simulink model "RealLifeTrainModel"  (R2024a)
settings: Solver=ode1  StartTime=0.0  StopTime=Inf  FixedStep=0.001  RelTol=1e-3
PostLoadFcn:
  | , if any(exist('dsrtsu_mdlpostloadfcn', 'file') ~= 0), dsrtsu_mdlpostloadfcn('Execute', bdroot); end,
InitFcn:
  | , if any(exist('rtifpga_mdlclblib', 'file') ~= 0), rtifpga_mdlclblib('Init', bdroot); end,
undefined symbols (not defined in the file): DiscIntNeverNeededParam
libraries: deeplib x29, svdutilitieslib x28, simulink x8, eeGeneralControl x8, rti1202lib_adc_class1 x6, rti1202serlib x5, spsEdgeDetectorLib x5, rtiemclib x2, rti1202lib_dac_class1 x1
(part 2 of 8)

== system RealLifeTrainModel/CommSystem ==
  Fload : Inport
  dFload : Inport  Port=2
  Fhyd : Inport  Port=3
  dFhyd : Inport  Port=4
  Pa : Inport  Port=5
  Pb : Inport  Port=6
  X : Inport  Port=7
  dX : Inport  Port=8
  Ref : Inport  Port=9
  last_action : Inport  Port=10
  last_action_rl : Inport  Port=11
  last_action_control : Inport  Port=12
  Enable : EnablePort
  Constant : Constant
  If4 : If  IfExpression=u1 & 1
  IncSubSystem : Subsystem  TreatAsAtomicUnit=on
  ScopeCounter : Scope
  SendMessageSystem : Subsystem  TreatAsAtomicUnit=on
  wires:
  last_action_control/1 -> SendMessageSystem/12(last_action_control)
  X/1 -> SendMessageSystem/7(X)
  dFhyd/1 -> SendMessageSystem/4(dFhyd)
  Fhyd/1 -> SendMessageSystem/3(Fhyd)
  If4/2 -> IncSubSystem/Action
  last_action_rl/1 -> SendMessageSystem/11(last_action_rl)
  last_action/1 -> SendMessageSystem/10(last_action)
  dFload/1 -> SendMessageSystem/2(dFload)
  Fload/1 -> SendMessageSystem/1(Fload)
  Pa/1 -> SendMessageSystem/5(Pa)
  dX/1 -> SendMessageSystem/8(dX)
  Pb/1 -> SendMessageSystem/6(Pb)
  If4/1 -> SendMessageSystem/Action
  Ref/1 -> SendMessageSystem/9(Ref)
  Constant/1 -> If4/1

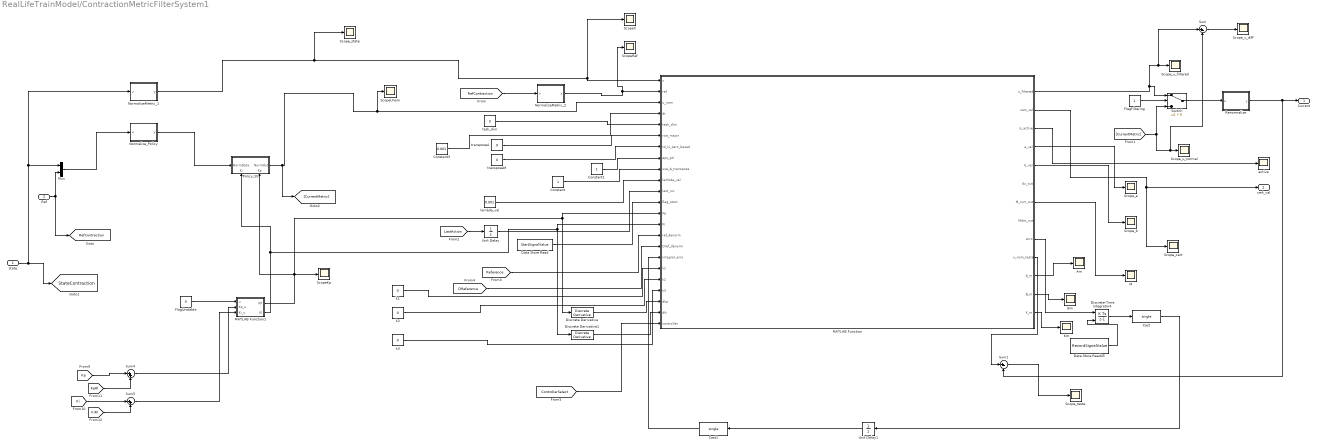
== system RealLifeTrainModel/ContractionMetricFilterSystem1 ==
  state : Inport
  Ref : Inport  Port=2
  Am : Scope
  Bm : Scope
  Cast : DataTypeConversion  OutDataTypeStr=single  SaturateOnIntegerOverflow=off  RndMeth=Floor
  Cast1 : DataTypeConversion  OutDataTypeStr=single  SaturateOnIntegerOverflow=off  RndMeth=Floor
  Constant : Constant
  Constant1 : Constant
  Constant3 : Constant  Value=0.001
  Data Store Read : DataStoreRead  DataStoreName=StartSignalValue  IndexOptions=Index vector (dialog)  Indices=1  OutputSizes=1
  Data Store Read45 : DataStoreRead  DataStoreName=RecordSignalValue  IndexOptions=Index vector (dialog)  Indices=1  OutputSizes=1
  Discrete Derivative : simulink/Discrete/Discrete Derivative  gainval=1.0  ICPrevScaledInput=0.0  OutMin=[]  OutMax=[]  OutDataType=fixdt(1, 16)  OutScaling=2^-10  DoSatur=off
  Discrete Derivative1 : simulink/Discrete/Discrete Derivative  gainval=1.0  ICPrevScaledInput=0.0  OutMin=[]  OutMax=[]  OutDataType=fixdt(1, 16)  OutScaling=2^-10  DoSatur=off
  Discrete-Time Integrator4 : DiscreteIntegrator  ExternalReset=falling  SampleTime=-1  ICPrevOutput=DiscIntNeverNeededParam  ICPrevScaledInput=DiscIntNeverNeededParam
  FlagFiltering : Constant
  FlagUnstable : Constant  Value=0
  Km : Scope
  M : Scope
  MATLAB Function : MATLAB Function  TreatAsAtomicUnit=on
  MATLAB Function1 : MATLAB Function  TreatAsAtomicUnit=on
  Mux : Mux  Inputs=2
  NormalizeMetric_1 : MATLAB Function  TreatAsAtomicUnit=on
  NormalizeMetric_2 : MATLAB Function  TreatAsAtomicUnit=on
  Normalize_Policy : MATLAB Function  TreatAsAtomicUnit=on
  Policy_SS : Subsystem
      settings: PortSchema="{\"entries\":[{\"content\":{\"sides\":[{\"content\":{\"connectorIds\":[\"In1\"]},\"type\":\"ConnectorPlacement.EquallySpacedRectSide\",\"uuid\":\"aff62fa4-063d-4c71-97b0-74a4cd3535bc\"},{\"content\":{\"connectorIds\":[\"Out1\"],\"side\":\"RIGHT\"},\"type\":\"ConnectorPlacement.EquallySpacedRectSide\",\"uuid\":\"01dd86b6-6835-48c6-94a2-7da686e8c645\"},{\"content\":{\"side\":\"TOP\"},\"type\":\"ConnectorPlacement.EquallySpacedRectSide\",\"uuid\":\"8b5720b6-3267-4312-8c98-f6d73204e352\"},{\"content\":{\"connectorIds\":[\"In2\",\"In3\"],\"side\":\"BOTTOM\"},\"type\":\"ConnectorPlacement.EquallySpacedRectSide\",\"uuid\":\"5afd0565-ca04-47d0-8ac2-f2d607cec9be\"}]},\"type\":\"ConnectorPlacement.EquallySpacedConnector\",\"uuid\":\"ef09f761-56e3-495c-a111-c24e12a3786f\"}],\"packageUris\":[\"http://schema.mathworks.com/mf0/Connector/R2020b\"],\"version\":\"1.0\"}"
  Renormalize : MATLAB Function  TreatAsAtomicUnit=on
  ScopeKp : Scope
  ScopeRef : Scope
  ScopeUnom : Scope
  ScopeX : Scope
  Scope_a : Scope
  Scope_b : Scope
  Scope_cert : Scope
  Scope_state : Scope
  Scope_teste : Scope
  Scope_u_diff : Scope
  Scope_u_filtered : Scope
  Scope_u_normal : Scope
  Sum : Sum  Inputs=|+-
  Sum1 : Sum  Inputs=|+-
  Sum4 : Sum  Inputs=|++
  Sum5 : Sum  Inputs=|++
  Switch : Switch  Criteria=u2 > Threshold  SaturateOnIntegerOverflow=off  InputSameDT=off
  Unit Delay : UnitDelay  SampleTime=-1  HasFrameUpgradeWarning=on
  Unit Delay1 : UnitDelay  SampleTime=-1  HasFrameUpgradeWarning=on
  active : Scope
  k1 : Constant  Value=0
  k2 : Constant  Value=0
  k3 : Constant  Value=0
  lambda_val : Constant  Value=0.001
  task_dim : Constant  Value=3
  transposeA : Constant  Value=0
  transposeM : Constant  Value=0
  Current : Outport
  cert_val : Outport  Port=2
  tag scope: RefContraction=global, StateContraction=global
  wires:
  Normalize_Policy/1(y) -> Policy_SS/1(NormData)
  Policy_SS/1(NormOut) -> [CurrentMetric], MATLAB Function/3(u_nom), ScopeUnom/1
  state/1 -> NormalizeMetric_1/1(u), Mux/1, [StateContraction]
  Ref/1 -> Mux/2, [RefContraction]
  Mux/1 -> Normalize_Policy/1(u)
  NormalizeMetric_1/1(y) -> Scope_state/1, ScopeX/1, MATLAB Function/1(x)
  [RefContraction] -> NormalizeMetric_2/1(u)
  NormalizeMetric_2/1(y) -> ScopeRef/1, MATLAB Function/2(ref)
  Renormalize/1(y) -> Sum1/2, Current/1
  MATLAB Function/2(cert_val) -> Scope_cert/1, cert_val/1
  MATLAB Function/3(is_active) -> active/1
  FlagFiltering/1 -> Switch/2
  MATLAB Function/1(u_filtered) -> Sum/1, Scope_u_filtered/1, Switch/1
  [CurrentMetric] -> Sum/2, Scope_u_normal/1, Switch/3
  Switch/1 -> Renormalize/1(u)
  Sum/1 -> Scope_u_diff/1
  MATLAB Function/4(a_val) -> Scope_a/1
  MATLAB Function/5(b_val) -> Scope_b/1
  Constant3/1 -> MATLAB Function/4(dt)
  task_dim/1 -> MATLAB Function/5(task_dim)
  transposeM/1 -> MATLAB Function/7(td_is_zero_based)
  lambda_val/1 -> MATLAB Function/10(lambda_val)
  [LastAction] -> Unit Delay/1
  Data Store Read/1 -> MATLAB Function/12(flag_start)
  MATLAB Function1/1(KP) -> MATLAB Function/13(Kp), Discrete Derivative/1, ScopeKp/1, Policy_SS/3(Kp)
  MATLAB Function1/2(KI) -> Policy_SS/2(Ki), MATLAB Function/14(Ki), Discrete Derivative1/1
  [Reference] -> MATLAB Function/15(ref_denorm)
  [DReference] -> MATLAB Function/16(Dref_denorm)
  Unit Delay/1 -> MATLAB Function/11(last_ixv)
  MATLAB Function/7(M_curr_out) -> M/1
  Data Store Read45/1 -> Discrete-Time Integrator4/2
  MATLAB Function/9(erro) -> Discrete-Time Integrator4/1
  Discrete-Time Integrator4/1 -> Cast/1
  Unit Delay1/1 -> Cast1/1
  Cast/1 -> Unit Delay1/1
  Cast1/1 -> MATLAB Function/17(integral_erro)
  MATLAB Function/10(u_nom_teste) -> Sum1/1
  Sum1/1 -> Scope_teste/1
  MATLAB Function/11(A_m) -> Am/1
  MATLAB Function/13(K_m) -> Km/1
  MATLAB Function/12(B_m) -> Bm/1
  Constant/1 -> MATLAB Function/9(use_A_transpose)
  Constant1/1 -> MATLAB Function/8(eps_pd)
  transposeA/1 -> MATLAB Function/6(row_major)
  k1/1 -> MATLAB Function/18(k1)
  k2/1 -> MATLAB Function/19(k2)
  k3/1 -> MATLAB Function/20(k3)
  [Kp] -> Sum4/1
  [Ki] -> Sum5/1
  [KiRl] -> Sum5/2
  [KpRl] -> Sum4/2
  Sum4/1 -> MATLAB Function1/2(Kp_s)
  Sum5/1 -> MATLAB Function1/3(Ki_s)
  FlagUnstable/1 -> MATLAB Function1/1(u)
  Discrete Derivative/1 -> MATLAB Function/21(dkp)
  Discrete Derivative1/1 -> MATLAB Function/22(dki)
  [ControllerSelect] -> MATLAB Function/23(controller)

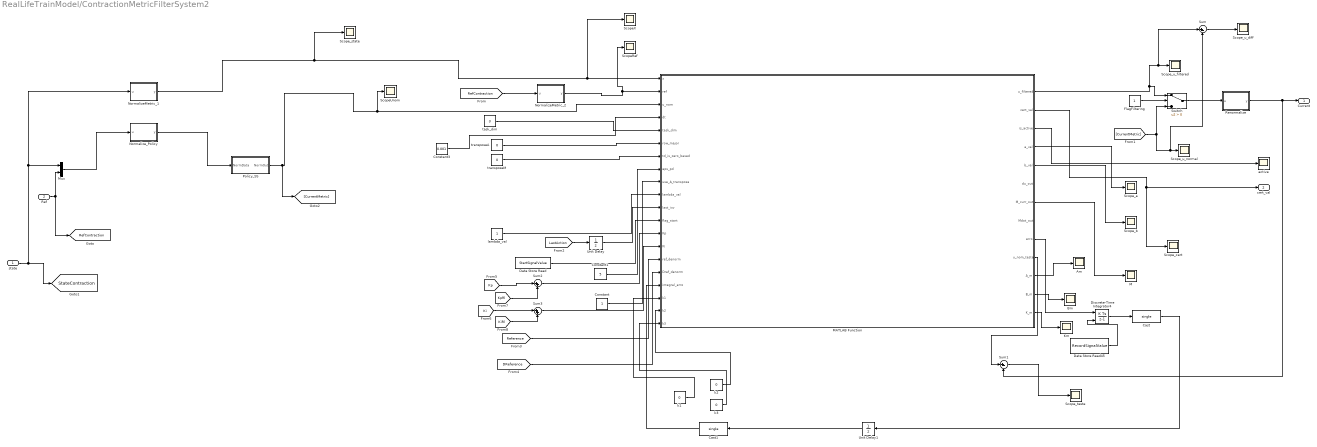
== system RealLifeTrainModel/ContractionMetricFilterSystem2 ==
  state : Inport
  Ref : Inport  Port=2
  Am : Scope
  Bm : Scope
  Cast : DataTypeConversion  OutDataTypeStr=single  SaturateOnIntegerOverflow=off  RndMeth=Floor
  Cast1 : DataTypeConversion  OutDataTypeStr=single  SaturateOnIntegerOverflow=off  RndMeth=Floor
  Constant : Constant
  Constant1 : Constant  Value=5
  Constant3 : Constant  Value=0.001
  Data Store Read : DataStoreRead  DataStoreName=StartSignalValue  IndexOptions=Index vector (dialog)  Indices=1  OutputSizes=1
  Data Store Read45 : DataStoreRead  DataStoreName=RecordSignalValue  IndexOptions=Index vector (dialog)  Indices=1  OutputSizes=1
  Discrete-Time Integrator4 : DiscreteIntegrator  ExternalReset=falling  SampleTime=-1  ICPrevOutput=DiscIntNeverNeededParam  ICPrevScaledInput=DiscIntNeverNeededParam
  FlagFiltering : Constant
  Km : Scope
  M : Scope
  MATLAB Function : MATLAB Function  TreatAsAtomicUnit=on
  Mux : Mux  Inputs=2
  NormalizeMetric_1 : MATLAB Function  TreatAsAtomicUnit=on
  NormalizeMetric_2 : MATLAB Function  TreatAsAtomicUnit=on
  Normalize_Policy : MATLAB Function  TreatAsAtomicUnit=on
  Policy_SS : Subsystem
  Renormalize : MATLAB Function  TreatAsAtomicUnit=on
  ScopeRef : Scope
  ScopeUnom : Scope
  ScopeX : Scope
  Scope_a : Scope
  Scope_b : Scope
  Scope_cert : Scope
  Scope_state : Scope
  Scope_teste : Scope
  Scope_u_diff : Scope
  Scope_u_filtered : Scope
  Scope_u_normal : Scope
  Sum : Sum  Inputs=|+-
  Sum1 : Sum  Inputs=|+-
  Sum2 : Sum  Inputs=|++
  Sum3 : Sum  Inputs=|++
  Switch : Switch  Criteria=u2 > Threshold  SaturateOnIntegerOverflow=off  InputSameDT=off
  Unit Delay : UnitDelay  SampleTime=-1  HasFrameUpgradeWarning=on
  Unit Delay1 : UnitDelay  SampleTime=-1  HasFrameUpgradeWarning=on
  active : Scope
  k1 : Constant  Value=0
  k2 : Constant  Value=0
  k3 : Constant  Value=0
  lambda_val : Constant
  task_dim : Constant  Value=3
  transposeA : Constant  Value=0
  transposeM : Constant  Value=0
  Current : Outport
  cert_val : Outport  Port=2
  tag scope: RefContraction=global, StateContraction=global
  wires:
  Normalize_Policy/1(y) -> Policy_SS/1(NormData)
  Policy_SS/1(NormOut) -> [CurrentMetric], MATLAB Function/3(u_nom), ScopeUnom/1
  state/1 -> NormalizeMetric_1/1(u), Mux/1, [StateContraction]
  Ref/1 -> Mux/2, [RefContraction]
  Mux/1 -> Normalize_Policy/1(u)
  NormalizeMetric_1/1(y) -> Scope_state/1, ScopeX/1, MATLAB Function/1(x)
  [RefContraction] -> NormalizeMetric_2/1(u)
  NormalizeMetric_2/1(y) -> ScopeRef/1, MATLAB Function/2(ref)
  Renormalize/1(y) -> Sum1/2, Current/1
  MATLAB Function/2(cert_val) -> Scope_cert/1, cert_val/1
  MATLAB Function/3(is_active) -> active/1
  FlagFiltering/1 -> Switch/2
  MATLAB Function/1(u_filtered) -> Sum/1, Scope_u_filtered/1, Switch/1
  [CurrentMetric] -> Sum/2, Scope_u_normal/1, Switch/3
  Switch/1 -> Renormalize/1(u)
  Sum/1 -> Scope_u_diff/1
  MATLAB Function/4(a_val) -> Scope_a/1
  MATLAB Function/5(b_val) -> Scope_b/1
  Constant3/1 -> MATLAB Function/4(dt)
  task_dim/1 -> MATLAB Function/5(task_dim)
  transposeM/1 -> MATLAB Function/7(td_is_zero_based)
  lambda_val/1 -> MATLAB Function/10(lambda_val)
  [LastAction] -> Unit Delay/1
  Data Store Read/1 -> MATLAB Function/12(flag_start)
  Sum2/1 -> MATLAB Function/13(Kp)
  Sum3/1 -> MATLAB Function/14(Ki)
  [Reference] -> MATLAB Function/15(ref_denorm)
  [DReference] -> MATLAB Function/16(Dref_denorm)
  [Kp] -> Sum2/1
  [Ki] -> Sum3/1
  [KpRl] -> Sum2/2
  [KiRl] -> Sum3/2
  Unit Delay/1 -> MATLAB Function/11(last_ixv)
  MATLAB Function/7(M_curr_out) -> M/1
  Data Store Read45/1 -> Discrete-Time Integrator4/2
  MATLAB Function/9(erro) -> Discrete-Time Integrator4/1
  Discrete-Time Integrator4/1 -> Cast/1
  Unit Delay1/1 -> Cast1/1
  Cast/1 -> Unit Delay1/1
  Cast1/1 -> MATLAB Function/17(integral_erro)
  MATLAB Function/10(u_nom_teste) -> Sum1/1
  Sum1/1 -> Scope_teste/1
  MATLAB Function/11(A_m) -> Am/1
  MATLAB Function/13(K_m) -> Km/1
  MATLAB Function/12(B_m) -> Bm/1
  Constant/1 -> MATLAB Function/9(use_A_transpose)
  Constant1/1 -> MATLAB Function/8(eps_pd)
  transposeA/1 -> MATLAB Function/6(row_major)
  k1/1 -> MATLAB Function/18(k1)
  k2/1 -> MATLAB Function/19(k2)
  k3/1 -> MATLAB Function/20(k3)

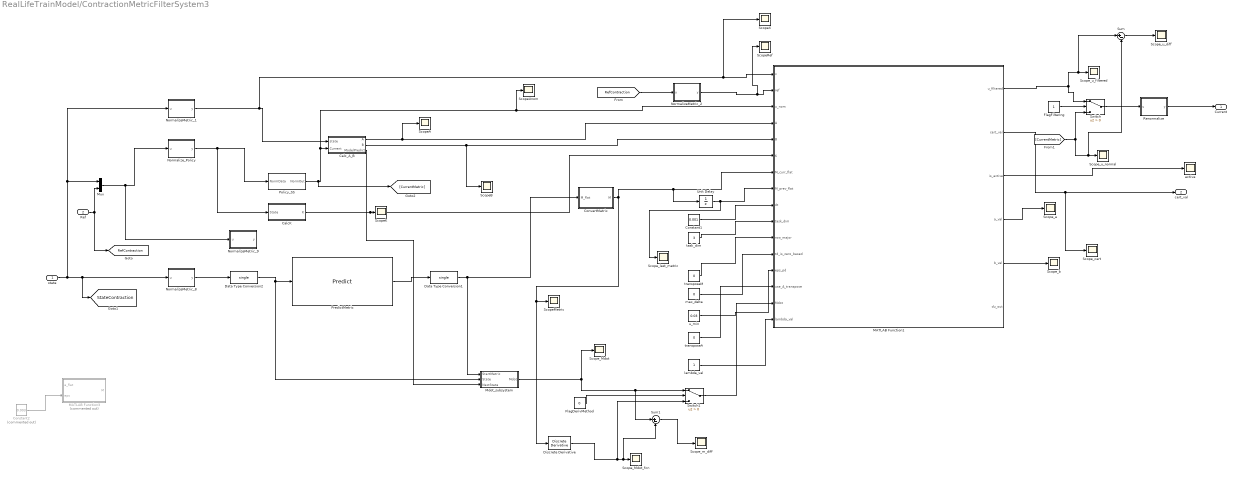
== system RealLifeTrainModel/ContractionMetricFilterSystem3 ==
  state : Inport
  Ref : Inport  Port=2
  CalcK : Subsystem
  Calc_A_B : Subsystem
  Constant1 : Constant  Value=0.001
  Constant2 : Constant  Commented=on  Value=0.003
  ConvertMatrix : MATLAB Function  TreatAsAtomicUnit=on
  Data Type Conversion1 : DataTypeConversion  OutDataTypeStr=single  SaturateOnIntegerOverflow=off  RndMeth=Floor
  Data Type Conversion2 : DataTypeConversion  OutDataTypeStr=single  SaturateOnIntegerOverflow=off  RndMeth=Floor
  Discrete Derivative : simulink/Discrete/Discrete Derivative  gainval=1.0  ICPrevScaledInput=0.0  OutMin=[]  OutMax=[]  OutDataType=fixdt(1, 16)  OutScaling=2^-10  DoSatur=off
  FlagDerivMethod : Constant  Value=0
  FlagFiltering : Constant
  MATLAB Function1 : MATLAB Function  TreatAsAtomicUnit=on
  MATLAB Function3 : MATLAB Function  Commented=on  TreatAsAtomicUnit=on
  Mdot_subsystem : Subsystem
  Mux : Mux  Inputs=2
  NormalizeMetric_1 : MATLAB Function  TreatAsAtomicUnit=on
  NormalizeMetric_2 : MATLAB Function  TreatAsAtomicUnit=on
  NormalizeMetric_8 : MATLAB Function  TreatAsAtomicUnit=on
  NormalizeMetric_9 : MATLAB Function  TreatAsAtomicUnit=on
  Normalize_Policy : MATLAB Function  TreatAsAtomicUnit=on
  Policy_SS : Subsystem
  PredictMetric : deeplib/Predict  Network=Network from MAT-file  NetworkFunction=squeezenet  NetworkFilePath=C:\Users\ic2d\Documents\GitHub\dSpace_Controllers_legged\metric.mat  MiniBatchSize=128  InputDataFormats={'input', 'BC';}  Predictions=on  Activations={}  ForceInterpretedSim=off  EnableDLNetwork=on  LastKnownNetworkFilePath='C:\Users\ic2d\Documents\GitHub\dSpace_Controllers_legged\metric.mat'  LastKnownNetworkTimeStamp=739864.429490740760229527950286865234375
  Renormalize : MATLAB Function  TreatAsAtomicUnit=on
  ScopeA : Scope
  ScopeB : Scope
  ScopeK : Scope
  ScopeMetric : Scope
  ScopeRef : Scope
  ScopeUnom : Scope
  ScopeX : Scope
  Scope_Mdot : Scope
  Scope_Mdot_fcn : Scope
  Scope_a : Scope
  Scope_b : Scope
  Scope_cert : Scope
  Scope_last_metric : Scope
  Scope_m_diff : Scope
  Scope_u_diff : Scope
  Scope_u_filtered : Scope
  Scope_u_normal : Scope
  Sum : Sum  Inputs=|+-
  Sum1 : Sum  Inputs=|+-
  Switch : Switch  Criteria=u2 > Threshold  SaturateOnIntegerOverflow=off  InputSameDT=off
  Switch1 : Switch  Criteria=u2 > Threshold  SaturateOnIntegerOverflow=off  InputSameDT=off
  Unit Delay : UnitDelay  SampleTime=-1  HasFrameUpgradeWarning=on
  active : Scope
  lambda_val : Constant
  max_delta : Constant  Value=0
  task_dim : Constant  Value=3
  transposeA : Constant  Value=0
  transposeM : Constant  Value=0
  u_min : Constant  Value=0.03
  Current : Outport
  cert_val : Outport  Port=2
  tag scope: RefContraction=global, StateContraction=global
  wires:
  Data Type Conversion2/1 -> Mdot_subsystem/2(State), PredictMetric/1
  Normalize_Policy/1(y) -> CalcK/1(State), Policy_SS/1(NormData)
  Policy_SS/1(NormOut) -> [CurrentMetric], ScopeUnom/1, MATLAB Function1/3(u_nom), Calc_A_B/2(Current)
  NormalizeMetric_8/1(y) -> Data Type Conversion2/1
  state/1 -> NormalizeMetric_1/1(u), Mux/1, [StateContraction], NormalizeMetric_8/1(u)
  Ref/1 -> Mux/2, [RefContraction]
  Mux/1 -> NormalizeMetric_9/1(u), Normalize_Policy/1(u)
  NormalizeMetric_1/1(y) -> ScopeX/1, MATLAB Function1/1(x), Calc_A_B/1(state)
  PredictMetric/1 -> Data Type Conversion1/1
  Constant1/1 -> MATLAB Function1/9(dt)
  u_min/1 -> MATLAB Function1/13(eps_pd)
  max_delta/1 -> MATLAB Function1/12(td_is_zero_based)
  lambda_val/1 -> MATLAB Function1/16(lambda_val)
  task_dim/1 -> MATLAB Function1/10(task_dim)
  [RefContraction] -> NormalizeMetric_2/1(u)
  NormalizeMetric_2/1(y) -> ScopeRef/1, MATLAB Function1/2(ref)
  Renormalize/1(y) -> Current/1
  MATLAB Function1/2(cert_val) -> Scope_cert/1, cert_val/1
  MATLAB Function1/3(is_active) -> active/1
  Data Type Conversion1/1 -> Mdot_subsystem/1(StartMetric), ConvertMatrix/1(M_flat)
  CalcK/1(K) -> MATLAB Function1/6(K), ScopeK/1
  Calc_A_B/1(A) -> MATLAB Function1/4(A), ScopeA/1
  FlagFiltering/1 -> Switch/2
  MATLAB Function1/1(u_filtered) -> Switch/1, Sum/1, Scope_u_filtered/1
  [CurrentMetric] -> Sum/2, Scope_u_normal/1, Switch/3
  Switch/1 -> Renormalize/1(u)
  Constant2/1 -> MATLAB Function3/2(eps)
  Sum/1 -> Scope_u_diff/1
  Calc_A_B/2(B) -> ScopeB/1, MATLAB Function1/5(B)
  MATLAB Function1/4(a_val) -> Scope_a/1
  MATLAB Function1/5(b_val) -> Scope_b/1
  Unit Delay/1 -> Scope_last_metric/1, MATLAB Function1/8(M_prev_flat)
  transposeA/1 -> MATLAB Function1/14(use_A_transpose)
  transposeM/1 -> MATLAB Function1/11(row_major)
  Calc_A_B/3(ModelPredict) -> Mdot_subsystem/3(NextState)
  Mdot_subsystem/1(Mdot) -> Scope_Mdot/1, Sum1/1, Switch1/1
  ConvertMatrix/1(M) -> Discrete Derivative/1, ScopeMetric/1, Unit Delay/1, MATLAB Function1/7(M_curr_flat)
  Discrete Derivative/1 -> Switch1/3, Sum1/2, Scope_Mdot_fcn/1
  Switch1/1 -> MATLAB Function1/15(Mdot)
  FlagDerivMethod/1 -> Switch1/2
  Sum1/1 -> Scope_m_diff/1

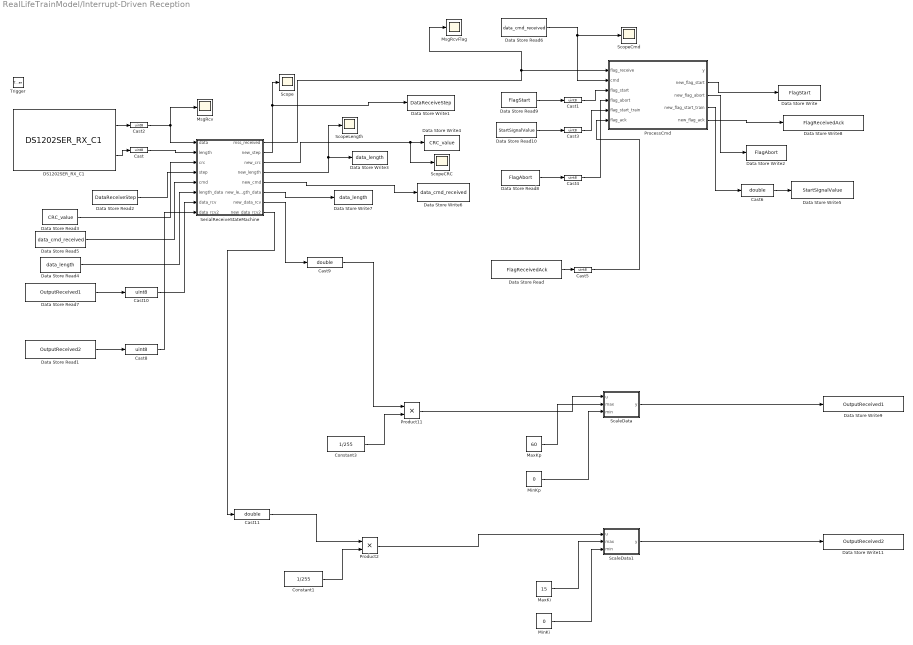
== system RealLifeTrainModel/Interrupt-Driven Reception ==
  Trigger : TriggerPort  TriggerType=function-call  VariantControl=Variant
  Cast{,1..5,8,10} (8 alike) : DataTypeConversion  OutDataTypeStr=uint8  SaturateOnIntegerOverflow=off  RndMeth=Floor
  Cast11 : DataTypeConversion  OutDataTypeStr=double  SaturateOnIntegerOverflow=off  RndMeth=Floor
  Cast6 : DataTypeConversion  OutDataTypeStr=double  SaturateOnIntegerOverflow=off  RndMeth=Floor
  Cast9 : DataTypeConversion  OutDataTypeStr=double  SaturateOnIntegerOverflow=off  RndMeth=Floor
  Constant1 : Constant  Value=1/255
  Constant3 : Constant  Value=1/255
  DS1202SER_RX_C1 : rti1202serlib/DS1202SER_RX_C1  Reserved1=[]  Reserved2=[]  Reserved3=[]  Reserved4=[]  DSProperties=struct('RTI',struct('IOBoardType',{{'DS1202','SER'}},'SlaveProcessor','NONE','Version',uint32(1),'BlockType',struct('isSLSource',uint8(1),'isSLSink',uint8(1),'isHWSource',uint8(0),'isHWSink',uint8(1),'isSetup',uint8(0),'isInline',uint8(1),'isNonInline',uint8(0),'isInterrupt',uint8(0),'isChannelwise',uint8(1)),'UnitType','GENSER','Identifier','RECEIVE','DialogType','ML','BlockSet','NONE'))  RTIBlockInterface=struct('BlockName',struct('Token',{{'DS1202SER_RX_C'}},'BlockParam',{{'ChannelNo'}}),'InputPortsWidth',int32(1),'InputPortsActive',0,'InputPortsDataType',{{'SS_UINT32'}},'InputPortsName',{{'NumBytes'}},'OutputPortsWidth',int32([7 1 1]),'OutputPortsActive',[1 1 0],'OutputPortsDataType',{{'SS_UINT8','SS_UINT32','SS_INT32'}},'OutputPortsName',{{'RXBytes','NumRXBytes','Status'}},'BlockDisplay',{{['Serial Receive'],'center'}},'IconTransparency','on','ParameterTunableNames',{{}},'InitLevel',2,'DialogFcn','guigenserreceive','MaskDescription',['To read data from the UART SW FIFO.'])  RTIBlockParameters=struct('BoardNo',{{1,'ON',[1 1]}},'ChannelNo',{{1,'ON',[1 2]}},'ChannelNumOf',{{2,'OFF',[]}},'ReceptionDataMode',{{1,'OFF',[]}},'ParamTunableMode',{{2,'OFF',[]}},'BytesRefNumOfT',{{'1','OFF',[1 inf]}},'BytesRefNumOfNT',{{'7','OFF',[1 inf]}},'BytesRefNumOfMax',{{'10','OFF',[1 inf]}},'BytesRefNumOfMode',{{0,'OFF',[]}},'BytesActNumOfMode',{{1,'OFF',[]}},'ReceptionStatusMode',{{0,'OFF',[]}},'FifoSizeDefault',{{64,'OFF',[]}},'TLCFileName',{{'rtigenserreceive','OFF',[]}})  RTISFcnParameters=struct('BoardNo','double','ChannelNo','double','ChannelNumOf','double','ReceptionDataMode','double','ParamTunableMode','double','BytesRefNumOfT','double','BytesRefNumOfNT','double','BytesRefNumOfMax','double','BytesRefNumOfMode','double','BytesActNumOfMode','double','ReceptionStatusMode','double','TLCFileName','char')  RTIBlockParaDefault=struct('BoardNo',1,'ChannelNo',1,'ChannelNumOf',2,'ReceptionDataMode',1,'ParamTunableMode',1,'BytesRefNumOfT',1,'BytesRefNumOfNT',1,'BytesRefNumOfMax',1,'BytesRefNumOfMode',0,'BytesActNumOfMode',1,'ReceptionStatusMode',1,'FifoSizeDefault',64,'TLCFileName','rtigenserreceive')
  Data Store Read : DataStoreRead  DataStoreName=FlagReceivedAck  IndexOptions=Index vector (dialog)  Indices=1  OutputSizes=1
  Data Store Read1 : DataStoreRead  DataStoreName=OutputReceived2  IndexOptions=Index vector (dialog)  Indices=1  OutputSizes=1
  Data Store Read10 : DataStoreRead  DataStoreName=StartSignalValue  IndexOptions=Index vector (dialog)  Indices=1  OutputSizes=1
  Data Store Read2 : DataStoreRead  DataStoreName=DataReceiveStep  IndexOptions=Index vector (dialog)  Indices=1  OutputSizes=1
  Data Store Read3 : DataStoreRead  DataStoreName=CRC_value  IndexOptions=Index vector (dialog)  Indices=1  OutputSizes=1
  Data Store Read4 : DataStoreRead  DataStoreName=data_length  IndexOptions=Index vector (dialog)  Indices=1  OutputSizes=1
  Data Store Read5 : DataStoreRead  DataStoreName=data_cmd_received  IndexOptions=Index vector (dialog)  Indices=1  OutputSizes=1
  Data Store Read6 : DataStoreRead  DataStoreName=data_cmd_received  IndexOptions=Index vector (dialog)  Indices=1  OutputSizes=1
  Data Store Read7 : DataStoreRead  DataStoreName=OutputReceived1  IndexOptions=Index vector (dialog)  Indices=1  OutputSizes=1
  Data Store Read8 : DataStoreRead  DataStoreName=FlagAbort  IndexOptions=Index vector (dialog)  Indices=1  OutputSizes=1
  Data Store Read9 : DataStoreRead  DataStoreName=FlagStart  IndexOptions=Index vector (dialog)  Indices=1  OutputSizes=1
  Data Store Write : DataStoreWrite  DataStoreName=FlagStart  IndexOptions=Index vector (dialog)  Indices=1  OutputSizes=1
  Data Store Write1 : DataStoreWrite  DataStoreName=DataReceiveStep  IndexOptions=Index vector (dialog)  Indices=1  OutputSizes=1
  Data Store Write11 : DataStoreWrite  DataStoreName=OutputReceived2  IndexOptions=Index vector (dialog)  Indices=1  OutputSizes=1
  Data Store Write2 : DataStoreWrite  DataStoreName=FlagAbort  IndexOptions=Index vector (dialog)  Indices=1  OutputSizes=1
  Data Store Write3 : DataStoreWrite  DataStoreName=data_length  IndexOptions=Index vector (dialog)  Indices=1  OutputSizes=1
  Data Store Write4 : DataStoreWrite  DataStoreName=CRC_value  IndexOptions=Index vector (dialog)  Indices=1  OutputSizes=1
  Data Store Write5 : DataStoreWrite  DataStoreName=StartSignalValue  IndexOptions=Index vector (dialog)  Indices=1  OutputSizes=1
  Data Store Write6 : DataStoreWrite  DataStoreName=data_cmd_received  IndexOptions=Index vector (dialog)  Indices=1  OutputSizes=1
  Data Store Write7 : DataStoreWrite  DataStoreName=data_length  IndexOptions=Index vector (dialog)  Indices=1  OutputSizes=1
  Data Store Write8 : DataStoreWrite  DataStoreName=FlagReceivedAck  IndexOptions=Index vector (dialog)  Indices=1  OutputSizes=1
  Data Store Write9 : DataStoreWrite  DataStoreName=OutputReceived1  IndexOptions=Index vector (dialog)  Indices=1  OutputSizes=1
  MaxKi : Constant  Value=15
  MaxKp : Constant  Value=60
  MinKi : Constant  Value=0
  MinKp : Constant  Value=0
  MsgRcv : Scope
  MsgRcvFlag : Scope
  ProcessCmd : MATLAB Function  TreatAsAtomicUnit=on
  Product11 : Product
  Product2 : Product
  ScaleData : MATLAB Function  TreatAsAtomicUnit=on
  ScaleData1 : MATLAB Function  TreatAsAtomicUnit=on
  Scope : Scope
  ScopeCRC : Scope
  ScopeCmd : Scope
  ScopeLength : Scope
  SerialReceiveStateMachine : MATLAB Function  TreatAsAtomicUnit=on
  wires:
  DS1202SER_RX_C1/1 -> Cast2/1
  SerialReceiveStateMachine/2(new_step) -> Scope/1, Data Store Write1/1
  Data Store Read2/1 -> SerialReceiveStateMachine/4(step)
  SerialReceiveStateMachine/4(new_length) -> ScopeLength/1, Data Store Write3/1
  SerialReceiveStateMachine/3(new_crc) -> ScopeCRC/1, Data Store Write4/1
  SerialReceiveStateMachine/1(mss_received) -> MsgRcvFlag/1, ProcessCmd/1(flag_receive)
  Data Store Read5/1 -> SerialReceiveStateMachine/5(cmd)
  Data Store Read4/1 -> SerialReceiveStateMachine/6(length_data)
  Data Store Read6/1 -> ProcessCmd/2(cmd), ScopeCmd/1
  SerialReceiveStateMachine/5(new_cmd) -> Data Store Write6/1
  SerialReceiveStateMachine/6(new_length_data) -> Data Store Write7/1
  ProcessCmd/2(new_flag_start) -> Data Store Write/1
  ProcessCmd/3(new_flag_abort) -> Data Store Write2/1
  ProcessCmd/4(new_flag_start_train) -> Cast6/1
  Data Store Read9/1 -> Cast1/1
  Data Store Read8/1 -> Cast4/1
  Data Store Read10/1 -> Cast3/1
  Data Store Read7/1 -> Cast10/1
  ProcessCmd/5(new_flag_ack) -> Data Store Write8/1
  Data Store Read/1 -> Cast5/1
  DS1202SER_RX_C1/2 -> Cast/1
  Cast/1 -> SerialReceiveStateMachine/2(length)
  Data Store Read3/1 -> SerialReceiveStateMachine/3(crc)
  Cast2/1 -> MsgRcv/1, SerialReceiveStateMachine/1(data)
  Cast1/1 -> ProcessCmd/3(flag_start)
  Cast3/1 -> ProcessCmd/5(flag_start_train)
  Cast4/1 -> ProcessCmd/4(flag_abort)
  Cast5/1 -> ProcessCmd/6(flag_ack)
  Cast6/1 -> Data Store Write5/1
  Constant3/1 -> Product11/2
  Cast9/1 -> Product11/1
  Cast10/1 -> SerialReceiveStateMachine/7(data_rcv)
  Data Store Read1/1 -> Cast8/1
  Cast8/1 -> SerialReceiveStateMachine/8(data_rcv2)
  SerialReceiveStateMachine/7(new_data_rcv) -> Cast9/1
  SerialReceiveStateMachine/8(new_data_rcv2) -> Cast11/1
  Cast11/1 -> Product2/1
  Constant1/1 -> Product2/2
  Product11/1 -> ScaleData/1(u)
  Product2/1 -> ScaleData1/1(u)
  MaxKp/1 -> ScaleData/2(max)
  MinKp/1 -> ScaleData/3(min)
  MaxKi/1 -> ScaleData1/2(max)
  MinKi/1 -> ScaleData1/3(min)
  ScaleData/1(y) -> Data Store Write9/1
  ScaleData1/1(y) -> Data Store Write11/1

== system RealLifeTrainModel/PolyDerivativeSubSystem1 ==
  Signal : Inport
  N : Inport  Port=2
  Constant : Constant  Value=0.001
  MATLAB Function : MATLAB Function  TreatAsAtomicUnit=on
  Mux : Mux  Inputs=40
  Unit Delay{1..39} (39 alike) : UnitDelay  SampleTime=-1  HasFrameUpgradeWarning=on
  dSignal : Outport
  ddSignal : Outport  Port=2
  dddSignal : Outport  Port=3
  wires:
  MATLAB Function/1(dx) -> dSignal/1
  Constant/1 -> MATLAB Function/2(Ts)
  Unit Delay12/1 -> Mux/5, Unit Delay13/1
  Unit Delay13/1 -> Mux/6, Unit Delay14/1
  Unit Delay9/1 -> Mux/2, Unit Delay10/1
  Unit Delay10/1 -> Mux/3, Unit Delay11/1
  Unit Delay11/1 -> Unit Delay12/1, Mux/4
  Signal/1 -> Mux/1, Unit Delay9/1
  Unit Delay15/1 -> Unit Delay16/1, Mux/8
  Unit Delay14/1 -> Mux/7, Unit Delay15/1
  Unit Delay16/1 -> Mux/9, Unit Delay1/1
  Unit Delay1/1 -> Unit Delay2/1, Mux/10
  Mux/1 -> MATLAB Function/1(k)
  Unit Delay2/1 -> Mux/11, Unit Delay3/1
  Unit Delay3/1 -> Mux/12, Unit Delay4/1
  Unit Delay4/1 -> Mux/13, Unit Delay5/1
  Unit Delay5/1 -> Mux/14, Unit Delay6/1
  Unit Delay6/1 -> Mux/15, Unit Delay7/1
  Unit Delay7/1 -> Unit Delay8/1, Mux/16
  Unit Delay8/1 -> Mux/17, Unit Delay17/1
  Unit Delay17/1 -> Mux/18, Unit Delay18/1
  Unit Delay18/1 -> Mux/19, Unit Delay19/1
  MATLAB Function/2(ddx) -> ddSignal/1
  MATLAB Function/3(dddx) -> dddSignal/1
  Unit Delay19/1 -> Unit Delay20/1, Mux/20
  Unit Delay20/1 -> Unit Delay21/1, Mux/21
  Unit Delay21/1 -> Unit Delay22/1, Mux/22
  Unit Delay22/1 -> Unit Delay23/1, Mux/23
  Unit Delay23/1 -> Unit Delay24/1, Mux/24
  Unit Delay24/1 -> Mux/25, Unit Delay25/1
  Unit Delay25/1 -> Unit Delay26/1, Mux/26
  Unit Delay26/1 -> Unit Delay27/1, Mux/27
  Unit Delay27/1 -> Unit Delay28/1, Mux/28
  Unit Delay28/1 -> Unit Delay29/1, Mux/29
  Unit Delay29/1 -> Unit Delay30/1, Mux/30
  Unit Delay30/1 -> Unit Delay31/1, Mux/31
  Unit Delay31/1 -> Unit Delay32/1, Mux/32
  Unit Delay32/1 -> Unit Delay33/1, Mux/33
  Unit Delay33/1 -> Unit Delay34/1, Mux/34
  Unit Delay34/1 -> Unit Delay35/1, Mux/35
  Unit Delay35/1 -> Unit Delay36/1, Mux/36
  Unit Delay36/1 -> Unit Delay37/1, Mux/37
  Unit Delay37/1 -> Unit Delay38/1, Mux/38
  Unit Delay38/1 -> Unit Delay39/1, Mux/39
  Unit Delay39/1 -> Mux/40
  N/1 -> MATLAB Function/3(n_points)

== system RealLifeTrainModel/PolyDerivativeSubSystem2 ==
  Signal : Inport
  N : Inport  Port=2
  Constant : Constant  Value=0.001
  MATLAB Function : MATLAB Function  TreatAsAtomicUnit=on
  Mux : Mux  Inputs=40
  Unit Delay{1..39} (39 alike) : UnitDelay  SampleTime=-1  HasFrameUpgradeWarning=on
  dSignal : Outport
  ddSignal : Outport  Port=2
  dddSignal : Outport  Port=3
  wires:
  MATLAB Function/1(dx) -> dSignal/1
  Constant/1 -> MATLAB Function/2(Ts)
  Unit Delay12/1 -> Mux/5, Unit Delay13/1
  Unit Delay13/1 -> Mux/6, Unit Delay14/1
  Unit Delay9/1 -> Mux/2, Unit Delay10/1
  Unit Delay10/1 -> Mux/3, Unit Delay11/1
  Unit Delay11/1 -> Unit Delay12/1, Mux/4
  Signal/1 -> Mux/1, Unit Delay9/1
  Unit Delay15/1 -> Unit Delay16/1, Mux/8
  Unit Delay14/1 -> Mux/7, Unit Delay15/1
  Unit Delay16/1 -> Mux/9, Unit Delay1/1
  Unit Delay1/1 -> Unit Delay2/1, Mux/10
  Mux/1 -> MATLAB Function/1(k)
  Unit Delay2/1 -> Mux/11, Unit Delay3/1
  Unit Delay3/1 -> Mux/12, Unit Delay4/1
  Unit Delay4/1 -> Mux/13, Unit Delay5/1
  Unit Delay5/1 -> Mux/14, Unit Delay6/1
  Unit Delay6/1 -> Mux/15, Unit Delay7/1
  Unit Delay7/1 -> Unit Delay8/1, Mux/16
  Unit Delay8/1 -> Mux/17, Unit Delay17/1
  Unit Delay17/1 -> Mux/18, Unit Delay18/1
  Unit Delay18/1 -> Mux/19, Unit Delay19/1
  MATLAB Function/2(ddx) -> ddSignal/1
  MATLAB Function/3(dddx) -> dddSignal/1
  Unit Delay19/1 -> Unit Delay20/1, Mux/20
  Unit Delay20/1 -> Unit Delay21/1, Mux/21
  Unit Delay21/1 -> Unit Delay22/1, Mux/22
  Unit Delay22/1 -> Unit Delay23/1, Mux/23
  Unit Delay23/1 -> Unit Delay24/1, Mux/24
  Unit Delay24/1 -> Mux/25, Unit Delay25/1
  Unit Delay25/1 -> Unit Delay26/1, Mux/26
  Unit Delay26/1 -> Unit Delay27/1, Mux/27
  Unit Delay27/1 -> Unit Delay28/1, Mux/28
  Unit Delay28/1 -> Unit Delay29/1, Mux/29
  Unit Delay29/1 -> Unit Delay30/1, Mux/30
  Unit Delay30/1 -> Unit Delay31/1, Mux/31
  Unit Delay31/1 -> Unit Delay32/1, Mux/32
  Unit Delay32/1 -> Unit Delay33/1, Mux/33
  Unit Delay33/1 -> Unit Delay34/1, Mux/34
  Unit Delay34/1 -> Unit Delay35/1, Mux/35
  Unit Delay35/1 -> Unit Delay36/1, Mux/36
  Unit Delay36/1 -> Unit Delay37/1, Mux/37
  Unit Delay37/1 -> Unit Delay38/1, Mux/38
  Unit Delay38/1 -> Unit Delay39/1, Mux/39
  Unit Delay39/1 -> Mux/40
  N/1 -> MATLAB Function/3(n_points)

== system RealLifeTrainModel/PolyDerivativeSubSystem3 ==
  Signal : Inport
  N : Inport  Port=2
  Constant : Constant  Value=0.001
  MATLAB Function : MATLAB Function  TreatAsAtomicUnit=on
  Mux : Mux  Inputs=40
  Unit Delay{1..39} (39 alike) : UnitDelay  SampleTime=-1  HasFrameUpgradeWarning=on
  dSignal : Outport
  ddSignal : Outport  Port=2
  dddSignal : Outport  Port=3
  wires:
  MATLAB Function/1(dx) -> dSignal/1
  Constant/1 -> MATLAB Function/2(Ts)
  Unit Delay12/1 -> Mux/5, Unit Delay13/1
  Unit Delay13/1 -> Mux/6, Unit Delay14/1
  Unit Delay9/1 -> Mux/2, Unit Delay10/1
  Unit Delay10/1 -> Mux/3, Unit Delay11/1
  Unit Delay11/1 -> Unit Delay12/1, Mux/4
  Signal/1 -> Mux/1, Unit Delay9/1
  Unit Delay15/1 -> Unit Delay16/1, Mux/8
  Unit Delay14/1 -> Mux/7, Unit Delay15/1
  Unit Delay16/1 -> Mux/9, Unit Delay1/1
  Unit Delay1/1 -> Unit Delay2/1, Mux/10
  Mux/1 -> MATLAB Function/1(k)
  Unit Delay2/1 -> Mux/11, Unit Delay3/1
  Unit Delay3/1 -> Mux/12, Unit Delay4/1
  Unit Delay4/1 -> Mux/13, Unit Delay5/1
  Unit Delay5/1 -> Mux/14, Unit Delay6/1
  Unit Delay6/1 -> Mux/15, Unit Delay7/1
  Unit Delay7/1 -> Unit Delay8/1, Mux/16
  Unit Delay8/1 -> Mux/17, Unit Delay17/1
  Unit Delay17/1 -> Mux/18, Unit Delay18/1
  Unit Delay18/1 -> Mux/19, Unit Delay19/1
  MATLAB Function/2(ddx) -> ddSignal/1
  MATLAB Function/3(dddx) -> dddSignal/1
  Unit Delay19/1 -> Unit Delay20/1, Mux/20
  Unit Delay20/1 -> Unit Delay21/1, Mux/21
  Unit Delay21/1 -> Unit Delay22/1, Mux/22
  Unit Delay22/1 -> Unit Delay23/1, Mux/23
  Unit Delay23/1 -> Unit Delay24/1, Mux/24
  Unit Delay24/1 -> Mux/25, Unit Delay25/1
  Unit Delay25/1 -> Unit Delay26/1, Mux/26
  Unit Delay26/1 -> Unit Delay27/1, Mux/27
  Unit Delay27/1 -> Unit Delay28/1, Mux/28
  Unit Delay28/1 -> Unit Delay29/1, Mux/29
  Unit Delay29/1 -> Unit Delay30/1, Mux/30
  Unit Delay30/1 -> Unit Delay31/1, Mux/31
  Unit Delay31/1 -> Unit Delay32/1, Mux/32
  Unit Delay32/1 -> Unit Delay33/1, Mux/33
  Unit Delay33/1 -> Unit Delay34/1, Mux/34
  Unit Delay34/1 -> Unit Delay35/1, Mux/35
  Unit Delay35/1 -> Unit Delay36/1, Mux/36
  Unit Delay36/1 -> Unit Delay37/1, Mux/37
  Unit Delay37/1 -> Unit Delay38/1, Mux/38
  Unit Delay38/1 -> Unit Delay39/1, Mux/39
  Unit Delay39/1 -> Mux/40
  N/1 -> MATLAB Function/3(n_points)

== system RealLifeTrainModel/PolyDerivativeSubSystem4 ==
  Signal : Inport
  Constant : Constant  Value=0.001
  MATLAB Function : MATLAB Function  TreatAsAtomicUnit=on
  Mux : Mux  Inputs=20
  Unit Delay{1..18} (18 alike) : UnitDelay  SampleTime=-1  HasFrameUpgradeWarning=on
  dSignal : Outport
  ddSignal : Outport  Port=2
  dddSignal : Outport  Port=3
  wires:
  MATLAB Function/1(dx) -> dSignal/1
  Constant/1 -> MATLAB Function/2(Ts)
  Unit Delay12/1 -> Mux/5, Unit Delay13/1
  Unit Delay13/1 -> Mux/6, Unit Delay14/1
  Unit Delay9/1 -> Mux/2, Unit Delay10/1
  Unit Delay10/1 -> Mux/3, Unit Delay11/1
  Unit Delay11/1 -> Unit Delay12/1, Mux/4
  Signal/1 -> Unit Delay9/1, Mux/1
  Unit Delay15/1 -> Unit Delay16/1, Mux/8
  Unit Delay14/1 -> Mux/7, Unit Delay15/1
  Unit Delay16/1 -> Unit Delay1/1, Mux/9
  Unit Delay1/1 -> Unit Delay2/1, Mux/10
  Mux/1 -> MATLAB Function/1(k)
  Unit Delay2/1 -> Unit Delay3/1, Mux/11
  Unit Delay3/1 -> Unit Delay4/1, Mux/12
  Unit Delay4/1 -> Unit Delay5/1, Mux/13
  Unit Delay5/1 -> Unit Delay6/1, Mux/14
  Unit Delay6/1 -> Unit Delay7/1, Mux/15
  Unit Delay7/1 -> Unit Delay8/1, Mux/16
  Unit Delay8/1 -> Unit Delay17/1, Mux/17
  Unit Delay17/1 -> Unit Delay18/1, Mux/18
  Unit Delay18/1 -> Mux/20, Mux/19
  MATLAB Function/2(ddx) -> ddSignal/1
  MATLAB Function/3(dddx) -> dddSignal/1

== system RealLifeTrainModel/PolyDerivativeSubSystem5 ==
  Signal : Inport
  N : Inport  Port=2
  Constant : Constant  Value=0.001
  MATLAB Function : MATLAB Function  TreatAsAtomicUnit=on
  Mux : Mux  Inputs=40
  Unit Delay{1..39} (39 alike) : UnitDelay  SampleTime=-1  HasFrameUpgradeWarning=on
  dSignal : Outport
  ddSignal : Outport  Port=2
  dddSignal : Outport  Port=3
  wires:
  MATLAB Function/1(dx) -> dSignal/1
  Constant/1 -> MATLAB Function/2(Ts)
  Unit Delay12/1 -> Mux/5, Unit Delay13/1
  Unit Delay13/1 -> Mux/6, Unit Delay14/1
  Unit Delay9/1 -> Mux/2, Unit Delay10/1
  Unit Delay10/1 -> Mux/3, Unit Delay11/1
  Unit Delay11/1 -> Unit Delay12/1, Mux/4
  Signal/1 -> Mux/1, Unit Delay9/1
  Unit Delay15/1 -> Unit Delay16/1, Mux/8
  Unit Delay14/1 -> Mux/7, Unit Delay15/1
  Unit Delay16/1 -> Mux/9, Unit Delay1/1
  Unit Delay1/1 -> Unit Delay2/1, Mux/10
  Mux/1 -> MATLAB Function/1(k)
  Unit Delay2/1 -> Mux/11, Unit Delay3/1
  Unit Delay3/1 -> Mux/12, Unit Delay4/1
  Unit Delay4/1 -> Mux/13, Unit Delay5/1
  Unit Delay5/1 -> Mux/14, Unit Delay6/1
  Unit Delay6/1 -> Mux/15, Unit Delay7/1
  Unit Delay7/1 -> Unit Delay8/1, Mux/16
  Unit Delay8/1 -> Mux/17, Unit Delay17/1
  Unit Delay17/1 -> Mux/18, Unit Delay18/1
  Unit Delay18/1 -> Mux/19, Unit Delay19/1
  MATLAB Function/2(ddx) -> ddSignal/1
  MATLAB Function/3(dddx) -> dddSignal/1
  Unit Delay19/1 -> Unit Delay20/1, Mux/20
  Unit Delay20/1 -> Unit Delay21/1, Mux/21
  Unit Delay21/1 -> Unit Delay22/1, Mux/22
  Unit Delay22/1 -> Unit Delay23/1, Mux/23
  Unit Delay23/1 -> Unit Delay24/1, Mux/24
  Unit Delay24/1 -> Mux/25, Unit Delay25/1
  Unit Delay25/1 -> Unit Delay26/1, Mux/26
  Unit Delay26/1 -> Unit Delay27/1, Mux/27
  Unit Delay27/1 -> Unit Delay28/1, Mux/28
  Unit Delay28/1 -> Unit Delay29/1, Mux/29
  Unit Delay29/1 -> Unit Delay30/1, Mux/30
  Unit Delay30/1 -> Unit Delay31/1, Mux/31
  Unit Delay31/1 -> Unit Delay32/1, Mux/32
  Unit Delay32/1 -> Unit Delay33/1, Mux/33
  Unit Delay33/1 -> Unit Delay34/1, Mux/34
  Unit Delay34/1 -> Unit Delay35/1, Mux/35
  Unit Delay35/1 -> Unit Delay36/1, Mux/36
  Unit Delay36/1 -> Unit Delay37/1, Mux/37
  Unit Delay37/1 -> Unit Delay38/1, Mux/38
  Unit Delay38/1 -> Unit Delay39/1, Mux/39
  Unit Delay39/1 -> Mux/40
  N/1 -> MATLAB Function/3(n_points)

== system RealLifeTrainModel/PolyDerivativeSubSystem6 ==
  Signal : Inport
  Constant : Constant  Value=0.001
  MATLAB Function : MATLAB Function  TreatAsAtomicUnit=on
  Mux : Mux  Inputs=20
  Unit Delay{1..18} (18 alike) : UnitDelay  SampleTime=-1  HasFrameUpgradeWarning=on
  dSignal : Outport
  ddSignal : Outport  Port=2
  dddSignal : Outport  Port=3
  wires:
  MATLAB Function/1(dx) -> dSignal/1
  Constant/1 -> MATLAB Function/2(Ts)
  Unit Delay12/1 -> Mux/5, Unit Delay13/1
  Unit Delay13/1 -> Mux/6, Unit Delay14/1
  Unit Delay9/1 -> Mux/2, Unit Delay10/1
  Unit Delay10/1 -> Mux/3, Unit Delay11/1
  Unit Delay11/1 -> Unit Delay12/1, Mux/4
  Signal/1 -> Unit Delay9/1, Mux/1
  Unit Delay15/1 -> Unit Delay16/1, Mux/8
  Unit Delay14/1 -> Mux/7, Unit Delay15/1
  Unit Delay16/1 -> Unit Delay1/1, Mux/9
  Unit Delay1/1 -> Unit Delay2/1, Mux/10
  Mux/1 -> MATLAB Function/1(k)
  Unit Delay2/1 -> Unit Delay3/1, Mux/11
  Unit Delay3/1 -> Unit Delay4/1, Mux/12
  Unit Delay4/1 -> Unit Delay5/1, Mux/13
  Unit Delay5/1 -> Unit Delay6/1, Mux/14
  Unit Delay6/1 -> Unit Delay7/1, Mux/15
  Unit Delay7/1 -> Unit Delay8/1, Mux/16
  Unit Delay8/1 -> Unit Delay17/1, Mux/17
  Unit Delay17/1 -> Unit Delay18/1, Mux/18
  Unit Delay18/1 -> Mux/20, Mux/19
  MATLAB Function/2(ddx) -> ddSignal/1
  MATLAB Function/3(dddx) -> dddSignal/1

== system RealLifeTrainModel/RTI Data ==
  RTI Data Store : Subsystem  Tag="struct('public',struct('sub',struct('name',{{'Teste_PID'}},'data',{{struct('TH',struct('thTaskInfo',struct('taskType',{'TIMER','HWINT','TMRINT','SWINT','GLINT'},'tasksNumOf',{1,1,0,0,0},'srcIds',{{'TIMERA'},{'UART_EVENTS_CH1_INT0'},{},{},{}},'taskNames',{{['Timer Task 1']},{'DS1202SER_INT_C1_I1'},{},{},{}})),'th_tc',struct('dataType',{'TASK','TASK'},'taskGroupId',{'',''},'taskGroupList',{{},{}},'taskSchedulingPolicy',{'FCFS','FCFS'},'taskType',{'TIMER','HWINT'},'blkh',{-1,'Teste_PID/DS1202SER_INT_C1_I1'},'srcId',{'TIMERA','UART_EVENTS_CH1_INT0'},'srcSgnName',{['Timer A interrupt'],['UART Ch1 RX SW FIFO interrupt']},'srcCpuName',{'',''},'taskName',{['Timer Task 1  [0.001] s'],'DS1202SER_INT_C1_I1'},'taskNameDisplayExt',{'',''},'smplTime',{0.001,0},'smplTimeOffs',{0,0},'hasFixedPriority',{0,0},'priority',{2,1},'hasFixedOvc',{0,0},'ovcType',{1,3},'ovcMax',{1,1}),'tc_th',struct('dataType',{'TASK','TASK'},'taskGroupId',{'',''},'taskGroupList',{{},{}},'taskSchedulingPolicy',{'FCFS','FCFS'},'taskType',{'TIMER','HWINT'},'blkh',{-1,'Teste_PID/DS1202SER_INT_C1_I1'},'srcId',{'TIMERA','UART_EVENTS_CH1_INT0'},'srcSgnName',{['Timer A interrupt'],['UART Ch1 RX SW FIFO interrupt']},'srcCpuName',{'',''},'taskName',{['Timer Task 1  [0.001] s'],'DS1202SER_INT_C1_I1'},'taskNameDisplayExt',{'',''},'smplTime',{0.001,0},'smplTimeOffs',{0,0},'hasFixedPriority',{0,0},'priority',{2,1},'hasFixedOvc',{0,0},'ovcType',{1,3},'ovcMax',{1,1}))}})),'private',struct('version',struct('dsVer',uint32(2)),'access',struct('type','Model','isPerm',1)))"  mask(RTI_DATA_STORE){}
      mask help:
      | RTI Data Store Block. This block is used by RTI to store internal model dependent data. Deleting this block will result in data loss.
      |
      | NEVER DELETE, COPY, OR MODIFY THIS BLOCK!
      mask Help:
      | RTI Data Store Block. This block is used by RTI to store internal model dependent data. Deleting this block will result in data loss.
      | 
      | NEVER DELETE, COPY, OR MODIFY THIS BLOCK!
      mask Display: text(0.5, 0.5, ' ', 'HorizontalAlignment', 'center');

== system RealLifeTrainModel/CommSystem/IncSubSystem ==
  Input : Inport
  Action Port : ActionPort  ActionPortLabel=else
  Constant : Constant
  Sum : Sum  Inputs=|++
  Out1 : Outport
  wires:
  Input/1 -> Sum/1
  Constant/1 -> Sum/2
  Sum/1 -> Out1/1

== system RealLifeTrainModel/CommSystem/SendMessageSystem ==
  Fload : Inport
  dFload : Inport  Port=2
  Fhyd : Inport  Port=3
  dFhyd : Inport  Port=4
  Pa : Inport  Port=5
  Pb : Inport  Port=6
  X : Inport  Port=7
  dX : Inport  Port=8
  Ref : Inport  Port=9
  last_action : Inport  Port=10
  last_action_rl : Inport  Port=11
  last_action_control : Inport  Port=12
  Action Port : ActionPort  ActionPortLabel=if(u1 & 1)
  AND1 : Logic  IconShape=distinctive  AllPortsSameDT=off  OutDataTypeStr=boolean
  AND2 : Logic  Inputs=3  IconShape=distinctive  AllPortsSameDT=off  OutDataTypeStr=boolean
  CancelSubsystem : Subsystem  TreatAsAtomicUnit=on
  Data Store Memory : DataStoreMemory  DataStoreName=CancelCounter  WriteAfterWriteMsg=warning  ShowAdditionalParam=off
  Data Store Memory1 : DataStoreMemory  DataStoreName=CancelLimit  WriteAfterWriteMsg=warning  InitialValue=7  ShowAdditionalParam=off
  Data Store Read : DataStoreRead  DataStoreName=StartSignalValue  IndexOptions=Index vector (dialog)  Indices=1  OutputSizes=1
  Data Store Read1 : DataStoreRead  DataStoreName=FlagReceivedAck  IndexOptions=Index vector (dialog)  Indices=1  OutputSizes=1
  Data Store Read2 : DataStoreRead  DataStoreName=CancelCounter  IndexOptions=Index vector (dialog)  Indices=1  OutputSizes=1
  Data Store Read3 : DataStoreRead  DataStoreName=CancelLimit  IndexOptions=Index vector (dialog)  Indices=1  OutputSizes=1
  Data Store Read6 : DataStoreRead  DataStoreName=FlagAbort  IndexOptions=Index vector (dialog)  Indices=1  OutputSizes=1
  Data Store Read7 : DataStoreRead  DataStoreName=StartSignalValue  IndexOptions=Index vector (dialog)  Indices=1  OutputSizes=1
  Data Store Read8 : DataStoreRead  DataStoreName=FlagAbort  IndexOptions=Index vector (dialog)  Indices=1  OutputSizes=1
  If Action Subsystem : Subsystem  TreatAsAtomicUnit=on
  If Action Subsystem1 : Subsystem  TreatAsAtomicUnit=on
  If2 : If  IfExpression="u1  == 1"
  If3 : If  IfExpression="u1  == 1"
  NOT1 : Logic  Operator=NOT  IconShape=distinctive  AllPortsSameDT=off  OutDataTypeStr=boolean
  NOT2 : Logic  Operator=NOT  IconShape=distinctive  AllPortsSameDT=off  OutDataTypeStr=boolean
  OR : Logic  Operator=OR  IconShape=distinctive  AllPortsSameDT=off  OutDataTypeStr=boolean
  ScopeFlagAck : Scope
  ScopeFlagStartTrain : Scope
  SendObs : Subsystem  TreatAsAtomicUnit=on
  SendObs1 : Subsystem  Commented=on  TreatAsAtomicUnit=on
  wires:
  Data Store Read6/1 -> OR/2
  OR/1 -> If2/1
  AND2/1 -> If3/1
  If3/1 -> SendObs/Action
  Data Store Read7/1 -> AND2/2
  If2/2 -> If Action Subsystem/Action
  If Action Subsystem/1(Out1) -> AND2/1
  Data Store Read8/1 -> NOT2/1
  AND1/1 -> OR/1
  Data Store Read1/1 -> ScopeFlagAck/1, NOT1/1
  NOT2/1 -> AND2/3
  NOT1/1 -> AND1/1
  If2/1 -> CancelSubsystem/Action
  Data Store Read/1 -> AND1/2, ScopeFlagStartTrain/1
  If3/2 -> If Action Subsystem1/Action
  Fload/1 -> SendObs/1(Fload)
  dFload/1 -> SendObs/2(dFload)
  Fhyd/1 -> SendObs/3(Fhyd)
  dFhyd/1 -> SendObs/4(dFhyd)
  Pa/1 -> SendObs/5(Pa)
  Pb/1 -> SendObs/6(Pb)
  X/1 -> SendObs/7(X)
  dX/1 -> SendObs/8(dX)
  Ref/1 -> SendObs/9(Ref)
  last_action/1 -> SendObs/10(last_action)
  last_action_rl/1 -> SendObs/11(last_action_rl)
  last_action_control/1 -> SendObs/12(last_action_control)
  Data Store Read2/1 -> CancelSubsystem/1(CancelCounter)
  Data Store Read3/1 -> CancelSubsystem/2(CancelLimit)

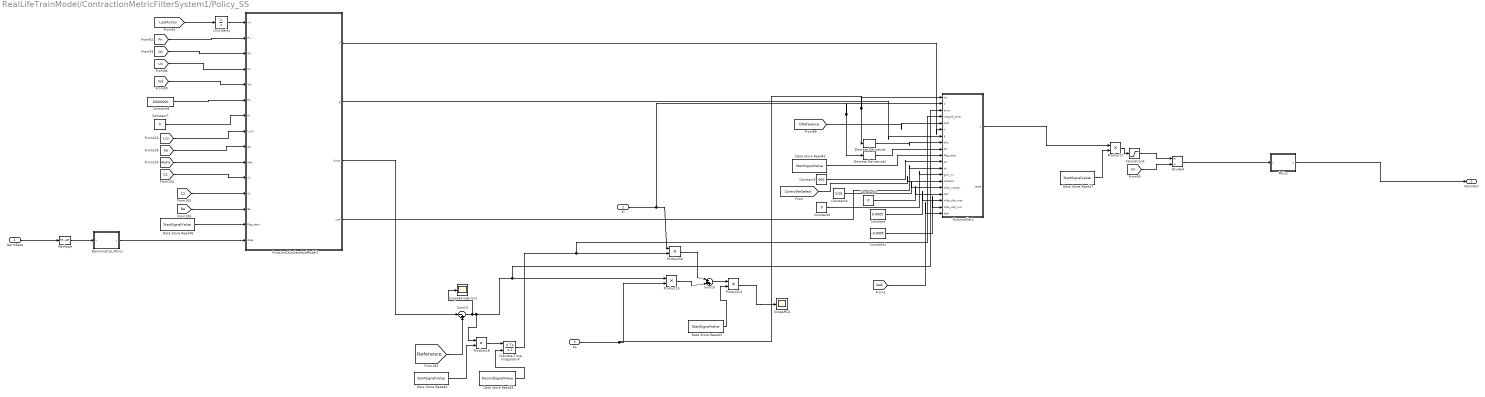
== system RealLifeTrainModel/ContractionMetricFilterSystem1/Policy_SS ==
  NormData : Inport
  Ki : Inport  Port=2
  Kp : Inport  Port=3
  Constant : Constant  Value=0.0005
  Constant1 : Constant  Value=-0.0005
  Constant3 : Constant  Value=0
  Constant4 : Constant  Value=0.05
  Constant5 : Constant  Value=600
  Constant6 : Constant  Value=0
  Constant7 : Constant  Value=0
  Constant8 : Constant  Value=16000000
  Data Store Read{42..44,46..47} (5 alike) : DataStoreRead  DataStoreName=StartSignalValue  IndexOptions=Index vector (dialog)  Indices=1  OutputSizes=1
  Data Store Read45 : DataStoreRead  DataStoreName=RecordSignalValue  IndexOptions=Index vector (dialog)  Indices=1  OutputSizes=1
  Denormalize_Policy : MATLAB Function  TreatAsAtomicUnit=on
  Discrete Derivative : simulink/Discrete/Discrete Derivative  gainval=1.0  ICPrevScaledInput=0.0  OutMin=[]  OutMax=[]  OutDataType=fixdt(1, 16)  OutScaling=2^-10  DoSatur=off
  Discrete Derivative1 : simulink/Discrete/Discrete Derivative  gainval=1.0  ICPrevScaledInput=0.0  OutMin=[]  OutMax=[]  OutDataType=fixdt(1, 16)  OutScaling=2^-10  DoSatur=off
  Discrete-Time Integrator4 : DiscreteIntegrator  ExternalReset=falling  SampleTime=-1  ICPrevOutput=DiscIntNeverNeededParam  ICPrevScaledInput=DiscIntNeverNeededParam
  Divide4 : Product  Inputs=*/
  FLcontroller1 : MATLAB Function  TreatAsAtomicUnit=on
  FunctionCalculateHydModel1 : MATLAB Function  TreatAsAtomicUnit=on
  Policy : MATLAB Function  TreatAsAtomicUnit=on
  Product{14..18} (5 alike) : Product
  Reshape : Reshape  OutputDimensionality=Row vector (2-D)  OutputDimensions=[8,1]
  Saturation5 : Saturate  UpperLimit=str2num(get_param('Teste_PID/Un','Value'))/str2num(get_param('Teste_PID/SaturationDivider','Value'))  LowerLimit=-str2num(get_param('Teste_PID/Un','Value'))/str2num(get_param('Teste_PID/SaturationDivider','Value'))
  ScopeForceError1 : Scope
  ScopePID1 : Scope
  Sum10 : Sum  Inputs=|+++
  Sum13 : Sum  Inputs=|-+
  Unit Delay : UnitDelay  SampleTime=-1  HasFrameUpgradeWarning=on
  NormOut : Outport
  wires:
  FunctionCalculateHydModel1/3(force) -> Sum13/1
  [Vpl] -> FunctionCalculateHydModel1/5(Vpl)
  Data Store Read45/1 -> Discrete-Time Integrator4/2
  Sum13/1 -> ScopeForceError1/1, FLcontroller1/3(error), Product15/1, Product18/1
  [Alpha] -> FunctionCalculateHydModel1/10(alfa)
  [C2] -> FunctionCalculateHydModel1/12(c2)
  [Be] -> FunctionCalculateHydModel1/13(Be)
  [Lcy] -> FunctionCalculateHydModel1/8(L_cyl)
  Data Store Read43/1 -> Product14/2
  [Ap] -> FunctionCalculateHydModel1/9(Aa)
  Product15/1 -> Sum10/2
  Data Store Read44/1 -> Product18/2
  Product18/1 -> Discrete-Time Integrator4/1
  [Reference] -> Sum13/2
  Constant8/1 -> FunctionCalculateHydModel1/6(Ps)
  Product14/1 -> ScopePID1/1
  Ki/1 -> Discrete Derivative1/1, FLcontroller1/2(ki), Product16/1
  Kp/1 -> Discrete Derivative/1, FLcontroller1/1(kp), Product15/2
  Saturation5/1 -> Divide4/1
  [Un] -> Divide4/2
  FLcontroller1/1(y) -> Product17/1
  Denormalize_Policy/1(y) -> FunctionCalculateHydModel1/15(data)
  Sum10/1 -> Product14/1
  [C1] -> FunctionCalculateHydModel1/11(c1)
  Discrete-Time Integrator4/1 -> FLcontroller1/4(integral_error), Product16/2
  [Pn] -> FunctionCalculateHydModel1/2(Pn)
  [LastAction] -> Unit Delay/1
  Constant7/1 -> FunctionCalculateHydModel1/7(Pt)
  Divide4/1 -> Policy/1(u)
  [Qn] -> FunctionCalculateHydModel1/3(Qn)
  Data Store Read47/1 -> Product17/2
  Product16/1 -> Sum10/1
  Product17/1 -> Saturation5/1
  [Un] -> FunctionCalculateHydModel1/4(Un)
  Data Store Read46/1 -> FunctionCalculateHydModel1/14(flag_start)
  NormData/1 -> Reshape/1
  Reshape/1 -> Denormalize_Policy/1(u)
  Unit Delay/1 -> FunctionCalculateHydModel1/1(ixv)
  Policy/1(y) -> NormOut/1
  [DReference] -> FLcontroller1/5(dref)
  Constant3/1 -> FLcontroller1/16(dist)
  Data Store Read42/1 -> FLcontroller1/10(flag_start)
  Constant/1 -> FLcontroller1/17(slide_dist_max)
  Constant1/1 -> FLcontroller1/18(slide_dist_min)
  [ControllerSelect] -> FLcontroller1/14(selector)
  Constant4/1 -> FLcontroller1/15(slide_margin)
  Constant5/1 -> FLcontroller1/11(psi)
  Constant6/1 -> FLcontroller1/13(gain_vc)
  FunctionCalculateHydModel1/2(g) -> FLcontroller1/7(g)
  FunctionCalculateHydModel1/1(f) -> FLcontroller1/6(h)
  Discrete Derivative/1 -> FLcontroller1/8(dkp)
  Discrete Derivative1/1 -> FLcontroller1/9(dki)
  FunctionCalculateHydModel1/4(xpd) -> FLcontroller1/12(dx)
  [leak] -> FLcontroller1/19(leak)
